simulink model "Rotational_Group4"  (R2024b)
settings: Solver=VariableStepAuto  StartTime=0.0  StopTime=Sim_Time  RelTol=1e-3
undefined symbols (not defined in the file): b, J, k
settings Model: Creator=ACER NITRO 5  LastModifiedBy=suave

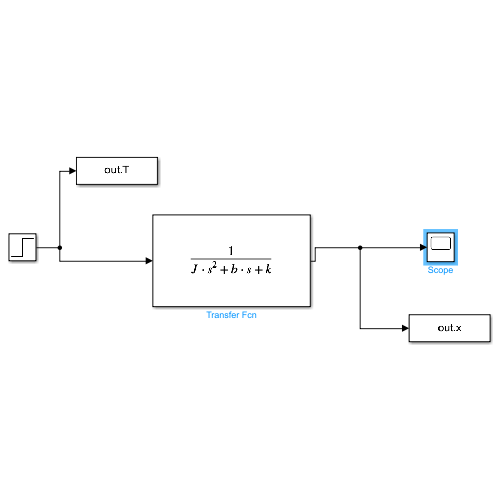
[thumbnail: Simulink's stored preview of the top-level diagram]
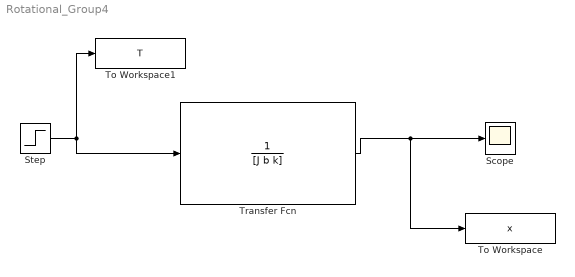
== system Rotational_Group4 ==
  Scope : Scope
  Step : Step  SampleTime=0
  To Workspace : ToWorkspace  VariableName=x  SaveFormat=Timeseries  SampleTime=-1
  To Workspace1 : ToWorkspace  VariableName=T  SaveFormat=Timeseries  SampleTime=-1
  Transfer Fcn : TransferFcn  Denominator=[J b k]
  wires:
  Step/1 -> To Workspace1/1, Transfer Fcn/1
  Transfer Fcn/1 -> To Workspace/1, Scope/1
